simulink library "csc_cac_coarse_acs_ctrl_lib"  (R2015b)
settings: Solver=ode45  StartTime=0.0  StopTime=10.0  RelTol=1e-3
values from neighbouring files (symbols this model uses):
  cac_alpha_gain_biprop_fire = 0.1    [csc_cac_coarse_acs_ctrl_init.m]
  cac_alpha_gain_coarse_only = 0.5    [csc_cac_coarse_acs_ctrl_init.m]
  cac_cg_offset_gain_compensation_x = [0 0 0 0 0 0 0 0 0 0 0 0 0 0 0 0 0 0 0 0 0]    [csc_cac_coarse_acs_ctrl_init.m]
  cac_cg_offset_gain_compensation_y = [0 0 0 0 0 0 0 0 0 0 0 0 0 0 0 0 0 0 0 0 0]    [csc_cac_coarse_acs_ctrl_init.m]
  cac_coarse_thruster_trq_x = cac_coarse_thruster_trq_x + cac_coarse_thruster_force*cac_coarse_trq_matx(cac_thruster_alloc_coarse_x_plus(i),1)    [csc_cac_coarse_acs_ctrl_prep.m]
  cac_coarse_thruster_trq_y = cac_coarse_thruster_trq_y + cac_coarse_thruster_force*cac_coarse_trq_matx(cac_thruster_alloc_coarse_y_plus(i),2)    [csc_cac_coarse_acs_ctrl_prep.m]
  cac_coarse_thruster_trq_z = cac_coarse_thruster_trq_z + cac_coarse_thruster_force*cac_coarse_trq_matx(cac_thruster_alloc_coarse_z_plus(i),3)    [csc_cac_coarse_acs_ctrl_prep.m]
  cac_rotx_deadband = 0.5*pi/180    (= 0.00872664625997)    [csc_cac_coarse_acs_ctrl_init.m]
  cac_rotx_deadband_minus = 0.5*pi/180    (= 0.00872664625997)    [csc_cac_coarse_acs_ctrl_init.m]
  cac_roty_deadband = 0.5*pi/180    (= 0.00872664625997)    [csc_cac_coarse_acs_ctrl_init.m]
  cac_roty_deadband_minus = 0.5*pi/180    (= 0.00872664625997)    [csc_cac_coarse_acs_ctrl_init.m]
  cac_rotz_deadband = 0.5*pi/180    (= 0.00872664625997)    [csc_cac_coarse_acs_ctrl_init.m]
  cac_rotz_deadband_minus = 0.5*pi/180    (= 0.00872664625997)    [csc_cac_coarse_acs_ctrl_init.m]
undefined symbols (not defined in the file or in its folder): emp_cg_wet_dry_range_x, emp_cg_wet_dry_range_y, emp_inertia_wet_dry, emp_mass_wet_dry
libraries: csu_ppd_phase_plane_distance_lib x3, simulink x1, util_info_lib x1, csu_ctp_coarse_thruster_pulse_command_new_lib x1
settings Model: Creator=Nilesh  LastModifiedBy=jimkaidy
settings DataIOCC: SaveFormat=Array
settings DebuggingCC: UnderspecifiedInitializationDetection=Classic  MergeDetectMultiDrivingBlocksExec=none  SolverPrmCheckMsg=warning  StateNameClashWarn=warning
settings HardwareCC: ProdBitPerPointer=32  ProdLargestAtomicFloat=None  ProdIntDivRoundTo=Undefined  ProdEndianess=Unspecified  ProdWordSize=32  ProdHWDeviceType=32-bit Generic
settings GRTTargetCC: GeneratePreprocessorConditionals=Disable all
settings ConfigComp: CovModelRefEnable=Off  CovSFcnEnable=off

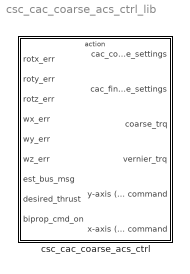
== system csc_cac_coarse_acs_ctrl_lib ==
  csc_cac_coarse_acs_ctrl : Subsystem

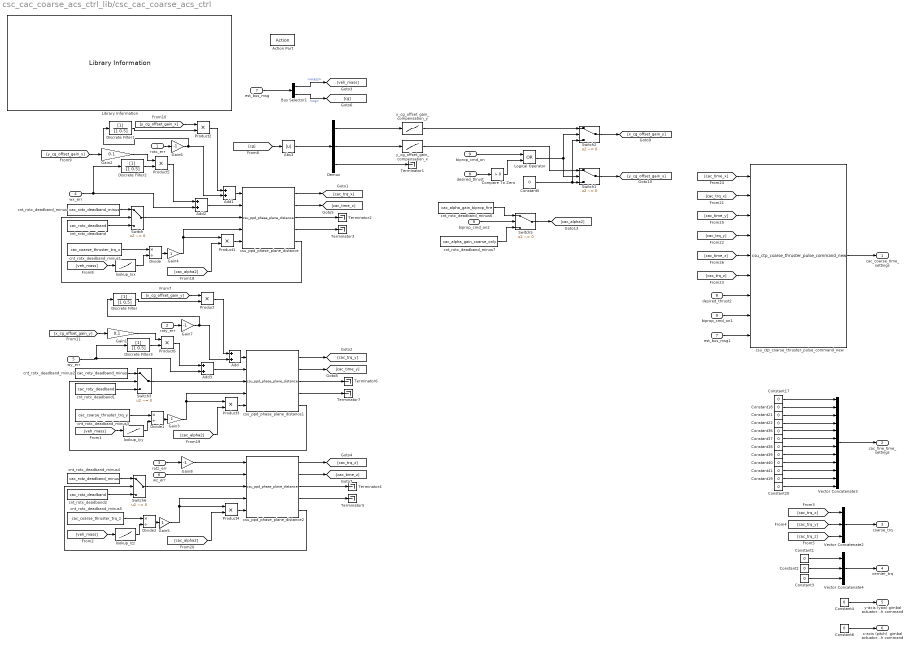
== system csc_cac_coarse_acs_ctrl_lib/csc_cac_coarse_acs_ctrl ==
  rotx_err : Inport
  roty_err : Inport  Port=2
  rotz_err : Inport  Port=3
  wx_err : Inport  Port=4
  wy_err : Inport  Port=5
  wz_err : Inport  Port=6
  est_bus_msg : Inport  Port=7
  desired_thrust : Inport  Port=8
  biprop_cmd_on : Inport  Port=9
  Action Port : ActionPort
  Abs3 : Abs
  Add{,1..3} (4 alike) : Sum
  Bus Selector1 : BusSelector  OutputSignals=mass,cg
  Compare To Zero : simulink/Logic and Bit Operations/Compare To Zero  relop=>  OutDataTypeStr=boolean
  Constant{1..4,6} (5 alike) : Constant  Value=0  OutDataTypeStr=int8
  Constant{17..22,36..41} (12 alike) : Constant  Value=0  OutDataTypeStr=uint8
  Constant5 : Constant  Value=0
  Demux : Demux  Outputs=3
  Discrete Filter{,1..3} (4 alike) : DiscreteFilter
  Divide : Product  Inputs=*/
  Divide1 : Product  Inputs=*/
  Divide2 : Product  Inputs=*/
  Gain1 : Gain  Gain=0.1
  Gain2 : Gain  Gain=0.1
  Gain3 : Gain
  Gain4 : Gain
  Gain5 : Gain
  Gain6 : Gain  Gain=-1
  Gain7 : Gain  Gain=-1
  Gain8 : Gain  Gain=-1
  Library Information : util_info_lib/Library Information  owner='Jim Kaidy <jimkaidy@moonexpress.com'
  Logical Operator : Logic  Operator=OR  AllPortsSameDT=off  OutDataTypeStr=boolean
  Product{,1..6} (7 alike) : Product
  Switch{,1..3,5..6} (6 alike) : Switch  Criteria=u2 ~= 0
  Terminator{1..7} (7 alike) : Terminator
  Vector Concatenate2 : Concatenate  NumInputs=3
  Vector Concatenate3 : Concatenate  NumInputs=12
  Vector Concatenate4 : Concatenate  NumInputs=3
  biprop_cmd_on1 : InportShadow  Port=9
  biprop_cmd_on2 : InportShadow  Port=9
  cnt_rotx_deadband : Constant  Value=cac_rotx_deadband
  cnt_rotx_deadband1 : Constant  Value=cac_roty_deadband
  cnt_rotx_deadband2 : Constant  Value=cac_rotz_deadband
  cnt_rotx_deadband_minus : Constant  Value=cac_rotx_deadband_minus
  cnt_rotx_deadband_minus1 : Constant  Value=cac_coarse_thruster_trq_x
  cnt_rotx_deadband_minus2 : Constant  Value=cac_roty_deadband_minus
  cnt_rotx_deadband_minus3 : Constant  Value=cac_coarse_thruster_trq_y
  cnt_rotx_deadband_minus4 : Constant  Value=cac_rotz_deadband_minus
  cnt_rotx_deadband_minus5 : Constant  Value=cac_coarse_thruster_trq_z
  cnt_rotx_deadband_minus6 : Constant  Value=cac_alpha_gain_biprop_fire
  cnt_rotx_deadband_minus7 : Constant  Value=cac_alpha_gain_coarse_only
  csu_ctp_coarse_thruster_pulse_command_new : csu_ctp_coarse_thruster_pulse_command_new_lib/csu_ctp_coarse_thruster_pulse_command_new
  csu_ppd_phase_plane_distance : csu_ppd_phase_plane_distance_lib/csu_ppd_phase_plane_distance
  csu_ppd_phase_plane_distance1 : csu_ppd_phase_plane_distance_lib/csu_ppd_phase_plane_distance
  csu_ppd_phase_plane_distance2 : csu_ppd_phase_plane_distance_lib/csu_ppd_phase_plane_distance
  desired_thrust2 : InportShadow  Port=8
  est_bus_msg1 : InportShadow  Port=7
  lookup_Ixx : Lookup  InputValues=emp_mass_wet_dry  Table=emp_inertia_wet_dry(1,:)
  lookup_Iyy : Lookup  InputValues=emp_mass_wet_dry  Table=emp_inertia_wet_dry(2,:)
  lookup_Izz : Lookup  InputValues=emp_mass_wet_dry  Table=emp_inertia_wet_dry(3,:)
  x_cg_offset_gain_compensation_y : Lookup  InputValues=emp_cg_wet_dry_range_x  Table=cac_cg_offset_gain_compensation_y
  y_cg_offset_gain_compensation_x : Lookup  InputValues=emp_cg_wet_dry_range_y  Table=cac_cg_offset_gain_compensation_x
  cac_coarse_time_settings : Outport
  cac_fine_time_settings : Outport  Port=2
  coarse_trq : Outport  Port=3
  vernier_trq : Outport  Port=4
  y-axis (yaw) gimbal actuator langth command : Outport  Port=5
  x-axis (pitch)  gimbal actuator langth command : Outport  Port=6
  wires:
  Vector Concatenate3/1 -> cac_fine_time_settings/1
  Constant3/1 -> Vector Concatenate4/3
  Constant2/1 -> Vector Concatenate4/2
  Constant1/1 -> Vector Concatenate4/1
  Vector Concatenate4/1 -> vernier_trq/1
  Constant38/1 -> Vector Concatenate3/7
  Constant39/1 -> Vector Concatenate3/8
  Constant37/1 -> Vector Concatenate3/6
  Constant36/1 -> Vector Concatenate3/5
  Constant40/1 -> Vector Concatenate3/9
  Constant41/1 -> Vector Concatenate3/10
  Constant22/1 -> Vector Concatenate3/4
  Constant21/1 -> Vector Concatenate3/3
  Constant19/1 -> Vector Concatenate3/11
  Constant18/1 -> Vector Concatenate3/2
  Constant20/1 -> Vector Concatenate3/12
  Constant17/1 -> Vector Concatenate3/1
  Vector Concatenate2/1 -> coarse_trq/1
  [cac_trq_z] -> Vector Concatenate2/3
  [cac_trq_y] -> Vector Concatenate2/2
  [cac_trq_x] -> Vector Concatenate2/1
  Divide/1 -> Gain4/1
  Switch/1 -> csu_ppd_phase_plane_distance/3
  cnt_rotx_deadband/1 -> Switch/3
  cnt_rotx_deadband_minus/1 -> Switch/1
  rotx_err/1 -> Gain6/1
  Switch3/1 -> csu_ppd_phase_plane_distance1/3
  roty_err/1 -> Gain7/1
  rotz_err/1 -> Gain8/1
  wz_err/1 -> csu_ppd_phase_plane_distance2/2
  Bus Selector1/1 -> [veh_mass]  "<mass>"
  [veh_mass] -> lookup_Ixx/1
  lookup_Ixx/1 -> Divide/2
  cnt_rotx_deadband_minus1/1 -> Divide/1
  cnt_rotx_deadband1/1 -> Switch3/3
  cnt_rotx_deadband_minus2/1 -> Switch3/1
  [veh_mass] -> lookup_Iyy/1
  lookup_Iyy/1 -> Divide1/2
  cnt_rotx_deadband_minus3/1 -> Divide1/1
  Divide1/1 -> Gain3/1
  Product3/1 -> csu_ppd_phase_plane_distance1/5
  Switch6/1 -> csu_ppd_phase_plane_distance2/3
  cnt_rotx_deadband2/1 -> Switch6/3
  cnt_rotx_deadband_minus4/1 -> Switch6/1
  csu_ppd_phase_plane_distance2/5 -> Switch6/2
  [veh_mass] -> lookup_Izz/1
  lookup_Izz/1 -> Divide2/2
  cnt_rotx_deadband_minus5/1 -> Divide2/1
  Divide2/1 -> Gain5/1
  Product4/1 -> csu_ppd_phase_plane_distance2/5
  csu_ppd_phase_plane_distance/1 -> [cac_trq_x]
  Gain4/1 -> Product1/1, csu_ppd_phase_plane_distance/4
  Gain8/1 -> csu_ppd_phase_plane_distance2/1
  csu_ppd_phase_plane_distance/2 -> [cac_time_x]
  csu_ppd_phase_plane_distance/5 -> Switch/2
  csu_ppd_phase_plane_distance1/1 -> [cac_trq_y]
  csu_ppd_phase_plane_distance1/2 -> [cac_time_y]
  csu_ppd_phase_plane_distance1/5 -> Switch3/2
  csu_ppd_phase_plane_distance2/1 -> [cac_trq_z]
  csu_ppd_phase_plane_distance2/2 -> [cac_time_z]
  Gain7/1 -> Add/2, Discrete Filter/1
  Product/1 -> Add/1
  Discrete Filter/1 -> Product/2
  Bus Selector1/2 -> [cg]  "<cg>"
  [x_cg_offset_gain_y] -> Product/1
  est_bus_msg/1 -> Bus Selector1/1
  [cg] -> Abs3/1
  Abs3/1 -> Demux/1
  Gain6/1 -> Discrete Filter1/1, Add1/2
  Product2/1 -> Add1/1
  Discrete Filter1/1 -> Product2/2
  [y_cg_offset_gain_x] -> Product2/1
  Add1/1 -> csu_ppd_phase_plane_distance/1
  csu_ppd_phase_plane_distance2/3 -> Terminator4/1
  csu_ppd_phase_plane_distance2/4 -> Terminator5/1
  Demux/2 -> y_cg_offset_gain_compensation_x/1
  Demux/3 -> Terminator1/1
  Constant5/1 -> Switch2/3, Switch1/3
  Logical Operator/1 -> Switch1/2, Switch2/2
  biprop_cmd_on/1 -> Logical Operator/1
  desired_thrust/1 -> Compare To Zero/1
  Compare To Zero/1 -> Logical Operator/2
  Demux/1 -> x_cg_offset_gain_compensation_y/1
  Switch2/1 -> [x_cg_offset_gain_y]
  Switch1/1 -> [y_cg_offset_gain_x]
  biprop_cmd_on2/1 -> Switch5/2
  cnt_rotx_deadband_minus6/1 -> Switch5/1
  cnt_rotx_deadband_minus7/1 -> Switch5/3
  Switch5/1 -> [cac_alpha2]
  [cac_alpha2] -> Product1/2
  Gain3/1 -> Product3/1, csu_ppd_phase_plane_distance1/4
  [cac_alpha2] -> Product3/2
  Gain5/1 -> Product4/1, csu_ppd_phase_plane_distance2/4
  [cac_alpha2] -> Product4/2
  x_cg_offset_gain_compensation_y/1 -> Switch2/1
  y_cg_offset_gain_compensation_x/1 -> Switch1/1
  Add/1 -> csu_ppd_phase_plane_distance1/1
  csu_ppd_phase_plane_distance1/3 -> Terminator6/1
  csu_ppd_phase_plane_distance1/4 -> Terminator7/1
  Product1/1 -> csu_ppd_phase_plane_distance/5
  csu_ppd_phase_plane_distance/3 -> Terminator2/1
  csu_ppd_phase_plane_distance/4 -> Terminator3/1
  wx_err/1 -> Discrete Filter2/1, Add2/2
  [y_cg_offset_gain_x] -> Gain2/1
  Discrete Filter2/1 -> Product5/2
  Gain2/1 -> Product5/1
  Product5/1 -> Add2/1
  Add2/1 -> csu_ppd_phase_plane_distance/2
  Gain1/1 -> Product6/1
  Add3/1 -> csu_ppd_phase_plane_distance1/2
  Product6/1 -> Add3/1
  wy_err/1 -> Discrete Filter3/1, Add3/2
  Discrete Filter3/1 -> Product6/2
  [x_cg_offset_gain_y] -> Gain1/1
  csu_ctp_coarse_thruster_pulse_command_new/1 -> cac_coarse_time_settings/1
  [cac_time_x] -> csu_ctp_coarse_thruster_pulse_command_new/1
  est_bus_msg1/1 -> csu_ctp_coarse_thruster_pulse_command_new/9
  [cac_time_z] -> csu_ctp_coarse_thruster_pulse_command_new/5
  [cac_trq_x] -> csu_ctp_coarse_thruster_pulse_command_new/2
  [cac_time_y] -> csu_ctp_coarse_thruster_pulse_command_new/3
  [cac_trq_z] -> csu_ctp_coarse_thruster_pulse_command_new/6
  [cac_trq_y] -> csu_ctp_coarse_thruster_pulse_command_new/4
  desired_thrust2/1 -> csu_ctp_coarse_thruster_pulse_command_new/7
  biprop_cmd_on1/1 -> csu_ctp_coarse_thruster_pulse_command_new/8
  Constant6/1 -> x-axis (pitch)  gimbal actuator langth command/1
  Constant4/1 -> y-axis (yaw) gimbal actuator langth command/1
